simulink model "HANcoder_E407_TTA_Controller_v4_5"  (R2018b)
settings: Solver=FixedStepDiscrete  StartTime=0.0  StopTime=1  FixedStep=0.01  RelTol=1e-3
PreLoadFcn:
  | librarySetup
  | eval([bdroot,'_startup']) %Calling [modelName]_startup.m
values from neighbouring files (symbols this model uses):
  Backup_Board = 0    [HANcoder_E407_TTA_Controller_v3_5_startup.m]    (also in HANcoder_E407_TTA_Controller_v4_6_startup.m; HANcoder_E407_TTA_Controller_v4_7_startup.m; HANcoder_E407_TTA_Controller_v4_startup.m)
  basic_cycle_duration_bc0 = TM_Reset_Board   + COMP_duration    (= 212)    [HANcoder_E407_TTA_Controller_v3_5_startup.m]    (also in HANcoder_E407_TTA_Controller_v4_6_startup.m; HANcoder_E407_TTA_Controller_v4_7_startup.m; HANcoder_E407_TTA_Controller_v4_startup.m)
  basic_cycle_duration_bc1 = TM_Reset_Var_bc1 + COMP_duration    (= 288)    [HANcoder_E407_TTA_Controller_v3_5_startup.m]    (also in HANcoder_E407_TTA_Controller_v4_6_startup.m = 332; HANcoder_E407_TTA_Controller_v4_7_startup.m = 372; HANcoder_E407_TTA_Controller_v4_startup.m = 332)
  comm_delay_estimation1 = round(comm_delay_measured1*hardware_granularity/frequency_IRQ)    [HANcoder_E407_TTA_Controller_v3_5_startup.m]    (also in HANcoder_E407_TTA_Controller_v4_6_startup.m; HANcoder_E407_TTA_Controller_v4_7_startup.m; HANcoder_E407_TTA_Controller_v4_startup.m)
  comm_delay_estimation2 = round(comm_delay_measured2*hardware_granularity/frequency_IRQ)    [HANcoder_E407_TTA_Controller_v3_5_startup.m]    (also in HANcoder_E407_TTA_Controller_v4_6_startup.m; HANcoder_E407_TTA_Controller_v4_7_startup.m; HANcoder_E407_TTA_Controller_v4_startup.m)
  COMM_Period = 40    [HANcoder_E407_TTA_Controller_v3_5_startup.m]    (also in HANcoder_E407_TTA_Controller_v4_6_startup.m; HANcoder_E407_TTA_Controller_v4_7_startup.m; HANcoder_E407_TTA_Controller_v4_startup.m)
  COMM_Phase1 = Simulink.Parameter    [HANcoder_E407_TTA_Controller_v3_5_startup.m]    (also in HANcoder_E407_TTA_Controller_v4_6_startup.m; HANcoder_E407_TTA_Controller_v4_7_startup.m; HANcoder_E407_TTA_Controller_v4_startup.m)
  COMM_Phase2 = Simulink.Parameter    [HANcoder_E407_TTA_Controller_v3_5_startup.m]    (also in HANcoder_E407_TTA_Controller_v4_6_startup.m; HANcoder_E407_TTA_Controller_v4_7_startup.m; HANcoder_E407_TTA_Controller_v4_startup.m)
  COMM_Phase_init1 = Simulink.Parameter    [HANcoder_E407_TTA_Controller_v3_5_startup.m]    (also in HANcoder_E407_TTA_Controller_v4_6_startup.m; HANcoder_E407_TTA_Controller_v4_7_startup.m; HANcoder_E407_TTA_Controller_v4_startup.m)
  COMM_Phase_init2 = Simulink.Parameter    [HANcoder_E407_TTA_Controller_v3_5_startup.m]    (also in HANcoder_E407_TTA_Controller_v4_6_startup.m; HANcoder_E407_TTA_Controller_v4_7_startup.m; HANcoder_E407_TTA_Controller_v4_startup.m)
  COMP_duration = 4    [HANcoder_E407_TTA_Controller_v3_5_startup.m]    (also in HANcoder_E407_TTA_Controller_v4_6_startup.m; HANcoder_E407_TTA_Controller_v4_7_startup.m; HANcoder_E407_TTA_Controller_v4_startup.m)
  Controller1_Board = 1    [HANcoder_E407_TTA_Controller_v3_5_startup.m]    (also in HANcoder_E407_TTA_Controller_v4_6_startup.m; HANcoder_E407_TTA_Controller_v4_7_startup.m; HANcoder_E407_TTA_Controller_v4_startup.m)
  Controller2_Board = 2    [HANcoder_E407_TTA_Controller_v3_5_startup.m]    (also in HANcoder_E407_TTA_Controller_v4_6_startup.m; HANcoder_E407_TTA_Controller_v4_7_startup.m; HANcoder_E407_TTA_Controller_v4_startup.m)
  Controller3_Board = 3    [HANcoder_E407_TTA_Controller_v3_5_startup.m]    (also in HANcoder_E407_TTA_Controller_v4_6_startup.m; HANcoder_E407_TTA_Controller_v4_7_startup.m; HANcoder_E407_TTA_Controller_v4_startup.m)
  delta_a_set = Simulink.Parameter    [HANcoder_E407_TTA_Controller_v3_5_startup.m]    (also in HANcoder_E407_TTA_Controller_v4_6_startup.m; HANcoder_E407_TTA_Controller_v4_7_startup.m; HANcoder_E407_TTA_Controller_v4_startup.m)
  delta_f_set = Simulink.Parameter    [HANcoder_E407_TTA_Controller_v3_5_startup.m]    (also in HANcoder_E407_TTA_Controller_v4_6_startup.m; HANcoder_E407_TTA_Controller_v4_7_startup.m; HANcoder_E407_TTA_Controller_v4_startup.m)
  delta_max = 1    [HANcoder_E407_TTA_Controller_v3_5_startup.m]    (also in HANcoder_E407_TTA_Controller_v4_6_startup.m; HANcoder_E407_TTA_Controller_v4_7_startup.m; HANcoder_E407_TTA_Controller_v4_startup.m)
  delta_min = -1    [HANcoder_E407_TTA_Controller_v3_5_startup.m]    (also in HANcoder_E407_TTA_Controller_v4_6_startup.m; HANcoder_E407_TTA_Controller_v4_7_startup.m; HANcoder_E407_TTA_Controller_v4_startup.m)
  delta_precision = 6    [HANcoder_E407_TTA_Controller_v3_5_startup.m]    (also in HANcoder_E407_TTA_Controller_v4_6_startup.m; HANcoder_E407_TTA_Controller_v4_7_startup.m; HANcoder_E407_TTA_Controller_v4_startup.m)
  e_width = 0.1    [HANcoder_E407_TTA_Controller_v3_5_startup.m]    (also in HANcoder_E407_TTA_Controller_v4_6_startup.m; HANcoder_E407_TTA_Controller_v4_7_startup.m; HANcoder_E407_TTA_Controller_v4_startup.m)
  frequency_IRQ = 100    [HANcoder_E407_2xCAN_TEST_startup.m]    (also in HANcoder_E407_TTA_Controller_v3_5_startup.m; HANcoder_E407_TTA_Controller_v4_6_startup.m; HANcoder_E407_TTA_Controller_v4_7_startup.m; HANcoder_E407_TTA_Controller_v4_startup.m)
  HANtuneOverride = Simulink.Parameter    [HANcoder_E407_2xCAN_TEST_startup.m]    (also in HANcoder_E407_TTA_Controller_v3_5_startup.m; HANcoder_E407_TTA_Controller_v4_6_startup.m; HANcoder_E407_TTA_Controller_v4_7_startup.m; HANcoder_E407_TTA_Controller_v4_startup.m)
  hardware_granularity = 1000000    [HANcoder_E407_2xCAN_TEST_startup.m]    (also in HANcoder_E407_TTA_Controller_v3_5_startup.m; HANcoder_E407_TTA_Controller_v4_6_startup.m; HANcoder_E407_TTA_Controller_v4_7_startup.m; HANcoder_E407_TTA_Controller_v4_startup.m)
  I_a = 2.25    [HANcoder_E407_TTA_Controller_v3_5_startup.m]    (also in HANcoder_E407_TTA_Controller_v4_6_startup.m; HANcoder_E407_TTA_Controller_v4_7_startup.m; HANcoder_E407_TTA_Controller_v4_startup.m)
  I_f = 2.25    [HANcoder_E407_TTA_Controller_v3_5_startup.m]    (also in HANcoder_E407_TTA_Controller_v4_6_startup.m; HANcoder_E407_TTA_Controller_v4_7_startup.m; HANcoder_E407_TTA_Controller_v4_startup.m)
  idle_time_init = basic_cycle_duration_bc0 + basic_cycle_duration_bc1    (= 500)    [HANcoder_E407_TTA_Controller_v3_5_startup.m]    (also in HANcoder_E407_TTA_Controller_v4_6_startup.m = 544; HANcoder_E407_TTA_Controller_v4_7_startup.m = 584; HANcoder_E407_TTA_Controller_v4_startup.m = 544)
  Input_Gen_Board = 4    [HANcoder_E407_TTA_Controller_v3_5_startup.m]    (also in HANcoder_E407_TTA_Controller_v4_6_startup.m; HANcoder_E407_TTA_Controller_v4_7_startup.m; HANcoder_E407_TTA_Controller_v4_startup.m)
  LA_Clock_Gr = 1    [HANcoder_E407_TTA_Controller_v3_5_startup.m]    (also in HANcoder_E407_TTA_Controller_v4_6_startup.m; HANcoder_E407_TTA_Controller_v4_7_startup.m; HANcoder_E407_TTA_Controller_v4_startup.m)
  LA_COMM_dly = 1    [HANcoder_E407_TTA_Controller_v3_5_startup.m]    (also in HANcoder_E407_TTA_Controller_v4_6_startup.m; HANcoder_E407_TTA_Controller_v4_7_startup.m; HANcoder_E407_TTA_Controller_v4_startup.m)
  LA_COMM_Err = 1    [HANcoder_E407_TTA_Controller_v3_5_startup.m]    (also in HANcoder_E407_TTA_Controller_v4_6_startup.m; HANcoder_E407_TTA_Controller_v4_7_startup.m; HANcoder_E407_TTA_Controller_v4_startup.m)
  LA_E_Desync = 1    [HANcoder_E407_TTA_Controller_v3_5_startup.m]    (also in HANcoder_E407_TTA_Controller_v4_6_startup.m; HANcoder_E407_TTA_Controller_v4_7_startup.m; HANcoder_E407_TTA_Controller_v4_startup.m)
  LA_MEX_Flag = 1    [HANcoder_E407_TTA_Controller_v3_5_startup.m]    (also in HANcoder_E407_TTA_Controller_v4_6_startup.m; HANcoder_E407_TTA_Controller_v4_7_startup.m; HANcoder_E407_TTA_Controller_v4_startup.m)
  LA_Task_Act = 1    [HANcoder_E407_TTA_Controller_v3_5_startup.m]    (also in HANcoder_E407_TTA_Controller_v4_6_startup.m; HANcoder_E407_TTA_Controller_v4_7_startup.m; HANcoder_E407_TTA_Controller_v4_startup.m)
  m_v = 100.0    (= 100)    [HANcoder_E407_TTA_Controller_v3_5_startup.m]    (also in HANcoder_E407_TTA_Controller_v4_6_startup.m; HANcoder_E407_TTA_Controller_v4_7_startup.m; HANcoder_E407_TTA_Controller_v4_startup.m)
  Master_Role = 1    [HANcoder_E407_TTA_Controller_v3_5_startup.m]    (also in HANcoder_E407_TTA_Controller_v4_6_startup.m; HANcoder_E407_TTA_Controller_v4_7_startup.m; HANcoder_E407_TTA_Controller_v4_startup.m)
  matrix_cycle_duration = basic_cycle_duration_bc0 + basic_cycle_duration_bc1    (= 500)    [HANcoder_E407_TTA_Controller_v3_5_startup.m]    (also in HANcoder_E407_TTA_Controller_v4_6_startup.m = 544; HANcoder_E407_TTA_Controller_v4_7_startup.m = 584; HANcoder_E407_TTA_Controller_v4_startup.m = 544)
  matrix_rows = 2    [HANcoder_E407_TTA_Controller_v3_5_startup.m]    (also in HANcoder_E407_TTA_Controller_v4_6_startup.m; HANcoder_E407_TTA_Controller_v4_7_startup.m; HANcoder_E407_TTA_Controller_v4_startup.m)
  max_desync = 15    [HANcoder_E407_TTA_Controller_v3_5_startup.m]    (also in HANcoder_E407_TTA_Controller_v4_6_startup.m; HANcoder_E407_TTA_Controller_v4_7_startup.m = 30; HANcoder_E407_TTA_Controller_v4_startup.m)
  max_num_msgs_CAN1 = 2^Tx_bit_number-1    (= 7)    [HANcoder_E407_TTA_Controller_v3_5_startup.m]    (also in HANcoder_E407_TTA_Controller_v4_6_startup.m = 15; HANcoder_E407_TTA_Controller_v4_7_startup.m = 15; HANcoder_E407_TTA_Controller_v4_startup.m)
  max_num_msgs_CAN2 = max_num_msgs_CAN1    (= 7)    [HANcoder_E407_TTA_Controller_v3_5_startup.m]    (also in HANcoder_E407_TTA_Controller_v4_6_startup.m = 15; HANcoder_E407_TTA_Controller_v4_7_startup.m = 15; HANcoder_E407_TTA_Controller_v4_startup.m)
  min_desync = (-1)*max_desync    (= -15)    [HANcoder_E407_TTA_Controller_v3_5_startup.m]    (also in HANcoder_E407_TTA_Controller_v4_6_startup.m; HANcoder_E407_TTA_Controller_v4_7_startup.m = -30; HANcoder_E407_TTA_Controller_v4_startup.m)
  OutControl1_ID = 23    [HANcoder_E407_TTA_Controller_v3_5_startup.m]    (also in HANcoder_E407_TTA_Controller_v4_6_startup.m; HANcoder_E407_TTA_Controller_v4_7_startup.m; HANcoder_E407_TTA_Controller_v4_startup.m)
  OutControl2_ID = 24    [HANcoder_E407_TTA_Controller_v3_5_startup.m]    (also in HANcoder_E407_TTA_Controller_v4_6_startup.m; HANcoder_E407_TTA_Controller_v4_7_startup.m; HANcoder_E407_TTA_Controller_v4_startup.m)
  OutEmulator_ID = 25    [HANcoder_E407_TTA_Controller_v3_5_startup.m]    (also in HANcoder_E407_TTA_Controller_v4_6_startup.m = 26; HANcoder_E407_TTA_Controller_v4_7_startup.m = 26; HANcoder_E407_TTA_Controller_v4_startup.m)
  OutMaster_ID = 25    [HANcoder_E407_TTA_Controller_v4_6_startup.m]    (also in HANcoder_E407_TTA_Controller_v4_7_startup.m; HANcoder_E407_TTA_Controller_v4_startup.m = 26)
  R_al = 0.10    (= 0.1)    [HANcoder_E407_TTA_Controller_v3_5_startup.m]    (also in HANcoder_E407_TTA_Controller_v4_6_startup.m; HANcoder_E407_TTA_Controller_v4_7_startup.m; HANcoder_E407_TTA_Controller_v4_startup.m)
  R_ar = 0.10    (= 0.1)    [HANcoder_E407_TTA_Controller_v3_5_startup.m]    (also in HANcoder_E407_TTA_Controller_v4_6_startup.m; HANcoder_E407_TTA_Controller_v4_7_startup.m; HANcoder_E407_TTA_Controller_v4_startup.m)
  R_fl = 0.10    (= 0.1)    [HANcoder_E407_TTA_Controller_v3_5_startup.m]    (also in HANcoder_E407_TTA_Controller_v4_6_startup.m; HANcoder_E407_TTA_Controller_v4_7_startup.m; HANcoder_E407_TTA_Controller_v4_startup.m)
  R_fr = 0.10    (= 0.1)    [HANcoder_E407_TTA_Controller_v3_5_startup.m]    (also in HANcoder_E407_TTA_Controller_v4_6_startup.m; HANcoder_E407_TTA_Controller_v4_7_startup.m; HANcoder_E407_TTA_Controller_v4_startup.m)
  script_run = Simulink.Parameter    [HANcoder_E407_TTA_Controller_v3_5_startup.m]    (also in HANcoder_E407_TTA_Controller_v4_6_startup.m; HANcoder_E407_TTA_Controller_v4_7_startup.m; HANcoder_E407_TTA_Controller_v4_startup.m)
  SensorValues_ID = 22    [HANcoder_E407_TTA_Controller_v3_5_startup.m]    (also in HANcoder_E407_TTA_Controller_v4_6_startup.m; HANcoder_E407_TTA_Controller_v4_7_startup.m; HANcoder_E407_TTA_Controller_v4_startup.m)
  SetValues_ID = 21    [HANcoder_E407_TTA_Controller_v3_5_startup.m]    (also in HANcoder_E407_TTA_Controller_v4_6_startup.m; HANcoder_E407_TTA_Controller_v4_7_startup.m; HANcoder_E407_TTA_Controller_v4_startup.m)
  Slave_Role = 2    [HANcoder_E407_TTA_Controller_v3_5_startup.m]    (also in HANcoder_E407_TTA_Controller_v4_6_startup.m; HANcoder_E407_TTA_Controller_v4_7_startup.m; HANcoder_E407_TTA_Controller_v4_startup.m)
  speed_k_d = Simulink.Parameter    [HANcoder_E407_TTA_Controller_v3_5_startup.m]    (also in HANcoder_E407_TTA_Controller_v4_6_startup.m; HANcoder_E407_TTA_Controller_v4_7_startup.m; HANcoder_E407_TTA_Controller_v4_startup.m)
  speed_k_i = Simulink.Parameter    [HANcoder_E407_TTA_Controller_v3_5_startup.m]    (also in HANcoder_E407_TTA_Controller_v4_6_startup.m; HANcoder_E407_TTA_Controller_v4_7_startup.m; HANcoder_E407_TTA_Controller_v4_startup.m)
  speed_k_p = Simulink.Parameter    [HANcoder_E407_TTA_Controller_v3_5_startup.m]    (also in HANcoder_E407_TTA_Controller_v4_6_startup.m; HANcoder_E407_TTA_Controller_v4_7_startup.m; HANcoder_E407_TTA_Controller_v4_startup.m)
  speed_max = 10    [HANcoder_E407_TTA_Controller_v3_5_startup.m]    (also in HANcoder_E407_TTA_Controller_v4_6_startup.m; HANcoder_E407_TTA_Controller_v4_7_startup.m; HANcoder_E407_TTA_Controller_v4_startup.m)
  speed_min = -10    [HANcoder_E407_TTA_Controller_v3_5_startup.m]    (also in HANcoder_E407_TTA_Controller_v4_6_startup.m; HANcoder_E407_TTA_Controller_v4_7_startup.m; HANcoder_E407_TTA_Controller_v4_startup.m)
  speed_precision = 3    [HANcoder_E407_TTA_Controller_v3_5_startup.m]    (also in HANcoder_E407_TTA_Controller_v4_6_startup.m; HANcoder_E407_TTA_Controller_v4_7_startup.m; HANcoder_E407_TTA_Controller_v4_startup.m)
  Sync_ID = 1    [HANcoder_E407_TTA_Controller_v3_5_startup.m]    (also in HANcoder_E407_TTA_Controller_v4_6_startup.m; HANcoder_E407_TTA_Controller_v4_7_startup.m; HANcoder_E407_TTA_Controller_v4_startup.m)
  tau_max = 5    [HANcoder_E407_TTA_Controller_v3_5_startup.m]    (also in HANcoder_E407_TTA_Controller_v4_6_startup.m; HANcoder_E407_TTA_Controller_v4_7_startup.m; HANcoder_E407_TTA_Controller_v4_startup.m)
  tau_min = -5    [HANcoder_E407_TTA_Controller_v3_5_startup.m]    (also in HANcoder_E407_TTA_Controller_v4_6_startup.m; HANcoder_E407_TTA_Controller_v4_7_startup.m; HANcoder_E407_TTA_Controller_v4_startup.m)
  tau_range = abs(tau_max) + abs(tau_min)    [HANcoder_E407_TTA_Controller_v3_5_startup.m]    (also in HANcoder_E407_TTA_Controller_v4_6_startup.m; HANcoder_E407_TTA_Controller_v4_7_startup.m; HANcoder_E407_TTA_Controller_v4_startup.m)
  theta_max = (speed_max/R_fr)*matrix_cycle_duration*frequency_IRQ/hardware_granularity    (= 5)    [HANcoder_E407_TTA_Controller_v3_5_startup.m]    (also in HANcoder_E407_TTA_Controller_v4_6_startup.m = 5.44; HANcoder_E407_TTA_Controller_v4_7_startup.m = 5.84; HANcoder_E407_TTA_Controller_v4_startup.m = 5.44)
  theta_min = (-1)*theta_max    (= -5)    [HANcoder_E407_TTA_Controller_v3_5_startup.m]    (also in HANcoder_E407_TTA_Controller_v4_6_startup.m = -5.44; HANcoder_E407_TTA_Controller_v4_7_startup.m = -5.84; HANcoder_E407_TTA_Controller_v4_startup.m = -5.44)
  theta_precision = 7-(fix(log2(theta_max))+1)    [HANcoder_E407_TTA_Controller_v3_5_startup.m]    (also in HANcoder_E407_TTA_Controller_v4_6_startup.m; HANcoder_E407_TTA_Controller_v4_7_startup.m; HANcoder_E407_TTA_Controller_v4_startup.m)
  Tl_a = 0.6    [HANcoder_E407_TTA_Controller_v3_5_startup.m]    (also in HANcoder_E407_TTA_Controller_v4_6_startup.m; HANcoder_E407_TTA_Controller_v4_7_startup.m; HANcoder_E407_TTA_Controller_v4_startup.m)
  Tl_f = 0.6    [HANcoder_E407_TTA_Controller_v3_5_startup.m]    (also in HANcoder_E407_TTA_Controller_v4_6_startup.m; HANcoder_E407_TTA_Controller_v4_7_startup.m; HANcoder_E407_TTA_Controller_v4_startup.m)
  TM_Check_Output_Control1 = TM_COMM_Output_Control1 + COMM_duration    (= 188)    [HANcoder_E407_TTA_Controller_v3_5_startup.m]    (also in HANcoder_E407_TTA_Controller_v4_6_startup.m; HANcoder_E407_TTA_Controller_v4_7_startup.m; HANcoder_E407_TTA_Controller_v4_startup.m)
  TM_Check_Output_Control2 = TM_COMM_Output_Control2 + COMM_duration    (= 232)    [HANcoder_E407_TTA_Controller_v3_5_startup.m]    (also in HANcoder_E407_TTA_Controller_v4_6_startup.m; HANcoder_E407_TTA_Controller_v4_7_startup.m; HANcoder_E407_TTA_Controller_v4_startup.m)
  TM_Check_Output_Emulator = TM_COMM_Output_Emulator + COMM_duration    (= 280)    [HANcoder_E407_TTA_Controller_v3_5_startup.m]    (also in HANcoder_E407_TTA_Controller_v4_6_startup.m = 320; HANcoder_E407_TTA_Controller_v4_7_startup.m = 360; HANcoder_E407_TTA_Controller_v4_startup.m = 320)
  TM_Check_Output_Emulator_2 = TM_Check_Output_Emulator + 2    (= 282)    [HANcoder_E407_TTA_Controller_v3_5_startup.m]    (also in HANcoder_E407_TTA_Controller_v4_6_startup.m = 322; HANcoder_E407_TTA_Controller_v4_7_startup.m = 362; HANcoder_E407_TTA_Controller_v4_startup.m = 322)
  TM_Check_Output_Emulator_3 = TM_Check_Output_Emulator_2 + 2    (= 324)    [HANcoder_E407_TTA_Controller_v4_6_startup.m]    (also in HANcoder_E407_TTA_Controller_v4_7_startup.m = 364; HANcoder_E407_TTA_Controller_v4_startup.m)
  TM_Check_Sensor_Values = TM_COMM_Sensor_Values + COMM_duration    (= 132)    [HANcoder_E407_TTA_Controller_v3_5_startup.m]    (also in HANcoder_E407_TTA_Controller_v4_6_startup.m; HANcoder_E407_TTA_Controller_v4_7_startup.m; HANcoder_E407_TTA_Controller_v4_startup.m)
  TM_Check_Sensor_Values_2 = TM_Check_Sensor_Values + 2    (= 134)    [HANcoder_E407_TTA_Controller_v3_5_startup.m]    (also in HANcoder_E407_TTA_Controller_v4_6_startup.m; HANcoder_E407_TTA_Controller_v4_7_startup.m; HANcoder_E407_TTA_Controller_v4_startup.m)
  TM_Check_Set_Values = TM_COMM_Set_Values + COMM_duration    (= 88)    [HANcoder_E407_TTA_Controller_v3_5_startup.m]    (also in HANcoder_E407_TTA_Controller_v4_6_startup.m; HANcoder_E407_TTA_Controller_v4_7_startup.m; HANcoder_E407_TTA_Controller_v4_startup.m)
  TM_Check_Set_Values_2 = TM_Check_Set_Values + 2    (= 90)    [HANcoder_E407_TTA_Controller_v3_5_startup.m]    (also in HANcoder_E407_TTA_Controller_v4_6_startup.m; HANcoder_E407_TTA_Controller_v4_7_startup.m; HANcoder_E407_TTA_Controller_v4_startup.m)
  TM_Check_Sync = TM_COMM_Sync   + COMM_duration    (= 40)    [HANcoder_E407_TTA_Controller_v3_5_startup.m]    (also in HANcoder_E407_TTA_Controller_v4_6_startup.m; HANcoder_E407_TTA_Controller_v4_7_startup.m; HANcoder_E407_TTA_Controller_v4_startup.m)
  TM_Check_TOuts = TM_Count_Vote3 + COMP_duration    (= 196)    [HANcoder_E407_TTA_Controller_v3_5_startup.m]    (also in HANcoder_E407_TTA_Controller_v4_6_startup.m; HANcoder_E407_TTA_Controller_v4_7_startup.m; HANcoder_E407_TTA_Controller_v4_startup.m)
  TM_Check_Vote1 = TM_COMM_Vote1  + COMM_duration    (= 92)    [HANcoder_E407_TTA_Controller_v3_5_startup.m]    (also in HANcoder_E407_TTA_Controller_v4_6_startup.m; HANcoder_E407_TTA_Controller_v4_7_startup.m; HANcoder_E407_TTA_Controller_v4_startup.m)
  TM_Check_Vote2 = TM_COMM_Vote2  + COMM_duration    (= 140)    [HANcoder_E407_TTA_Controller_v3_5_startup.m]    (also in HANcoder_E407_TTA_Controller_v4_6_startup.m; HANcoder_E407_TTA_Controller_v4_7_startup.m; HANcoder_E407_TTA_Controller_v4_startup.m)
  TM_Check_Vote2_2 = TM_Check_Vote2 + 2    (= 142)    [HANcoder_E407_TTA_Controller_v3_5_startup.m]    (also in HANcoder_E407_TTA_Controller_v4_6_startup.m; HANcoder_E407_TTA_Controller_v4_7_startup.m; HANcoder_E407_TTA_Controller_v4_startup.m)
  TM_Check_Vote3 = TM_COMM_Vote3  + COMM_duration    (= 188)    [HANcoder_E407_TTA_Controller_v3_5_startup.m]    (also in HANcoder_E407_TTA_Controller_v4_6_startup.m; HANcoder_E407_TTA_Controller_v4_7_startup.m; HANcoder_E407_TTA_Controller_v4_startup.m)
  TM_COMM_Output_Control1 = TM_Velocity + COMP_duration    (= 148)    [HANcoder_E407_TTA_Controller_v3_5_startup.m]    (also in HANcoder_E407_TTA_Controller_v4_6_startup.m; HANcoder_E407_TTA_Controller_v4_7_startup.m; HANcoder_E407_TTA_Controller_v4_startup.m)
  TM_COMM_Output_Control2 = TM_Check_Output_Control1 + COMP_duration    (= 192)    [HANcoder_E407_TTA_Controller_v3_5_startup.m]    (also in HANcoder_E407_TTA_Controller_v4_6_startup.m; HANcoder_E407_TTA_Controller_v4_7_startup.m; HANcoder_E407_TTA_Controller_v4_startup.m)
  TM_COMM_Output_Emulator = TM_TMR + COMP_duration    (= 240)    [HANcoder_E407_TTA_Controller_v3_5_startup.m]    (also in HANcoder_E407_TTA_Controller_v4_6_startup.m = 280; HANcoder_E407_TTA_Controller_v4_7_startup.m = 320; HANcoder_E407_TTA_Controller_v4_startup.m = 280)
  TM_COMM_Output_Master = TM_Check_Output_Control2 + COMM_duration    (= 272)    [HANcoder_E407_TTA_Controller_v4_6_startup.m]    (also in HANcoder_E407_TTA_Controller_v4_7_startup.m; HANcoder_E407_TTA_Controller_v4_startup.m)
  TM_COMM_Sensor_Values = TM_Check_Set_Values + COMP_duration    (= 92)    [HANcoder_E407_TTA_Controller_v3_5_startup.m]    (also in HANcoder_E407_TTA_Controller_v4_6_startup.m; HANcoder_E407_TTA_Controller_v4_7_startup.m; HANcoder_E407_TTA_Controller_v4_startup.m)
  TM_COMM_Set_Values = TM_Update_LT + COMP_duration    (= 48)    [HANcoder_E407_TTA_Controller_v3_5_startup.m]    (also in HANcoder_E407_TTA_Controller_v4_6_startup.m; HANcoder_E407_TTA_Controller_v4_7_startup.m; HANcoder_E407_TTA_Controller_v4_startup.m)
  TM_COMM_Sync = basic_cycle_start    (= 0)    [HANcoder_E407_TTA_Controller_v3_5_startup.m]    (also in HANcoder_E407_TTA_Controller_v4_6_startup.m; HANcoder_E407_TTA_Controller_v4_7_startup.m; HANcoder_E407_TTA_Controller_v4_startup.m)
  TM_COMM_Vote1 = TM_Vote_Dec    + COMP_duration    (= 52)    [HANcoder_E407_TTA_Controller_v3_5_startup.m]    (also in HANcoder_E407_TTA_Controller_v4_6_startup.m; HANcoder_E407_TTA_Controller_v4_7_startup.m; HANcoder_E407_TTA_Controller_v4_startup.m)
  TM_COMM_Vote2 = TM_Count_Vote1 + COMP_duration    (= 100)    [HANcoder_E407_TTA_Controller_v3_5_startup.m]    (also in HANcoder_E407_TTA_Controller_v4_6_startup.m; HANcoder_E407_TTA_Controller_v4_7_startup.m; HANcoder_E407_TTA_Controller_v4_startup.m)
  TM_COMM_Vote3 = TM_Count_Vote2 + COMP_duration    (= 148)    [HANcoder_E407_TTA_Controller_v3_5_startup.m]    (also in HANcoder_E407_TTA_Controller_v4_6_startup.m; HANcoder_E407_TTA_Controller_v4_7_startup.m; HANcoder_E407_TTA_Controller_v4_startup.m)
  TM_Count_Vote1 = TM_Check_Vote1 + COMP_duration    (= 96)    [HANcoder_E407_TTA_Controller_v3_5_startup.m]    (also in HANcoder_E407_TTA_Controller_v4_6_startup.m; HANcoder_E407_TTA_Controller_v4_7_startup.m; HANcoder_E407_TTA_Controller_v4_startup.m)
  TM_Count_Vote2 = TM_Check_Vote2 + COMP_duration    (= 144)    [HANcoder_E407_TTA_Controller_v3_5_startup.m]    (also in HANcoder_E407_TTA_Controller_v4_6_startup.m; HANcoder_E407_TTA_Controller_v4_7_startup.m; HANcoder_E407_TTA_Controller_v4_startup.m)
  TM_Count_Vote3 = TM_Check_Vote3 + COMP_duration    (= 192)    [HANcoder_E407_TTA_Controller_v3_5_startup.m]    (also in HANcoder_E407_TTA_Controller_v4_6_startup.m; HANcoder_E407_TTA_Controller_v4_7_startup.m; HANcoder_E407_TTA_Controller_v4_startup.m)
  TM_Data_bc0 = TM_COMM_Sync    (= 0)    [HANcoder_E407_TTA_Controller_v3_5_startup.m]    (also in HANcoder_E407_TTA_Controller_v4_6_startup.m; HANcoder_E407_TTA_Controller_v4_7_startup.m; HANcoder_E407_TTA_Controller_v4_startup.m)
  TM_Data_bc1 = TM_Data_bc0(1:4)    [HANcoder_E407_TTA_Controller_v3_5_startup.m]    (also in HANcoder_E407_TTA_Controller_v4_6_startup.m; HANcoder_E407_TTA_Controller_v4_7_startup.m; HANcoder_E407_TTA_Controller_v4_startup.m)
  TM_New_Master = TM_Check_TOuts + COMP_duration    (= 200)    [HANcoder_E407_TTA_Controller_v3_5_startup.m]    (also in HANcoder_E407_TTA_Controller_v4_6_startup.m; HANcoder_E407_TTA_Controller_v4_7_startup.m; HANcoder_E407_TTA_Controller_v4_startup.m)
  TM_Reset_Board = TM_Reset_Var   + COMP_duration    (= 208)    [HANcoder_E407_TTA_Controller_v3_5_startup.m]    (also in HANcoder_E407_TTA_Controller_v4_6_startup.m; HANcoder_E407_TTA_Controller_v4_7_startup.m; HANcoder_E407_TTA_Controller_v4_startup.m)
  TM_Reset_Var = TM_New_Master  + COMP_duration    (= 204)    [HANcoder_E407_TTA_Controller_v3_5_startup.m]    (also in HANcoder_E407_TTA_Controller_v4_6_startup.m; HANcoder_E407_TTA_Controller_v4_7_startup.m; HANcoder_E407_TTA_Controller_v4_startup.m)
  TM_Reset_Var_bc1 = TM_Check_Output_Emulator + COMP_duration    (= 284)    [HANcoder_E407_TTA_Controller_v3_5_startup.m]    (also in HANcoder_E407_TTA_Controller_v4_6_startup.m = 328; HANcoder_E407_TTA_Controller_v4_7_startup.m = 368; HANcoder_E407_TTA_Controller_v4_startup.m = 328)
  TM_Reset_Var_bc1_2 = TM_Reset_Var_bc1 + 2    (= 286)    [HANcoder_E407_TTA_Controller_v3_5_startup.m]    (also in HANcoder_E407_TTA_Controller_v4_6_startup.m = 330; HANcoder_E407_TTA_Controller_v4_7_startup.m = 370; HANcoder_E407_TTA_Controller_v4_startup.m = 330)
  TM_Steer = TM_Check_Sensor_Values + COMP_duration    (= 136)    [HANcoder_E407_TTA_Controller_v3_5_startup.m]    (also in HANcoder_E407_TTA_Controller_v4_6_startup.m; HANcoder_E407_TTA_Controller_v4_7_startup.m; HANcoder_E407_TTA_Controller_v4_startup.m)
  TM_TMR = TM_Check_Output_Control2 + COMP_duration    (= 236)    [HANcoder_E407_TTA_Controller_v3_5_startup.m]    (also in HANcoder_E407_TTA_Controller_v4_6_startup.m = 276; HANcoder_E407_TTA_Controller_v4_7_startup.m = 316; HANcoder_E407_TTA_Controller_v4_startup.m = 276)
  TM_TMR_2 = TM_TMR + 1    (= 237)    [HANcoder_E407_TTA_Controller_v3_5_startup.m]    (also in HANcoder_E407_TTA_Controller_v4_6_startup.m = 277; HANcoder_E407_TTA_Controller_v4_7_startup.m = 317; HANcoder_E407_TTA_Controller_v4_startup.m = 277)
  TM_TMR_3 = TM_TMR + 3    (= 239)    [HANcoder_E407_TTA_Controller_v3_5_startup.m]    (also in HANcoder_E407_TTA_Controller_v4_6_startup.m = 279; HANcoder_E407_TTA_Controller_v4_7_startup.m = 319; HANcoder_E407_TTA_Controller_v4_startup.m = 279)
  TM_Torque = TM_Steer + COMP_duration    (= 140)    [HANcoder_E407_TTA_Controller_v3_5_startup.m]    (also in HANcoder_E407_TTA_Controller_v4_6_startup.m; HANcoder_E407_TTA_Controller_v4_7_startup.m; HANcoder_E407_TTA_Controller_v4_startup.m)
  TM_Type_bc0 = COMM    (= 0)    [HANcoder_E407_TTA_Controller_v3_5_startup.m]    (also in HANcoder_E407_TTA_Controller_v4_6_startup.m; HANcoder_E407_TTA_Controller_v4_7_startup.m; HANcoder_E407_TTA_Controller_v4_startup.m)
  TM_Type_bc1 = TM_Type_bc0(1:4)    [HANcoder_E407_TTA_Controller_v3_5_startup.m]    (also in HANcoder_E407_TTA_Controller_v4_6_startup.m; HANcoder_E407_TTA_Controller_v4_7_startup.m; HANcoder_E407_TTA_Controller_v4_startup.m)
  TM_Update_LT = TM_Check_Sync  + COMP_duration    (= 44)    [HANcoder_E407_TTA_Controller_v3_5_startup.m]    (also in HANcoder_E407_TTA_Controller_v4_6_startup.m; HANcoder_E407_TTA_Controller_v4_7_startup.m; HANcoder_E407_TTA_Controller_v4_startup.m)
  TM_Update_LT_2 = TM_Update_LT   + 2    (= 46)    [HANcoder_E407_TTA_Controller_v3_5_startup.m]    (also in HANcoder_E407_TTA_Controller_v4_6_startup.m; HANcoder_E407_TTA_Controller_v4_7_startup.m; HANcoder_E407_TTA_Controller_v4_startup.m)
  TM_Velocity = TM_Torque + COMP_duration    (= 144)    [HANcoder_E407_TTA_Controller_v3_5_startup.m]    (also in HANcoder_E407_TTA_Controller_v4_6_startup.m; HANcoder_E407_TTA_Controller_v4_7_startup.m; HANcoder_E407_TTA_Controller_v4_startup.m)
  TM_Vote_Dec = TM_Update_LT   + COMP_duration    (= 48)    [HANcoder_E407_TTA_Controller_v3_5_startup.m]    (also in HANcoder_E407_TTA_Controller_v4_6_startup.m; HANcoder_E407_TTA_Controller_v4_7_startup.m; HANcoder_E407_TTA_Controller_v4_startup.m)
  TM_Vote_Dec_2 = TM_Vote_Dec    + 2    (= 50)    [HANcoder_E407_TTA_Controller_v3_5_startup.m]    (also in HANcoder_E407_TTA_Controller_v4_6_startup.m; HANcoder_E407_TTA_Controller_v4_7_startup.m; HANcoder_E407_TTA_Controller_v4_startup.m)
  torque_a_k_d = Simulink.Parameter    [HANcoder_E407_TTA_Controller_v3_5_startup.m]    (also in HANcoder_E407_TTA_Controller_v4_6_startup.m; HANcoder_E407_TTA_Controller_v4_7_startup.m; HANcoder_E407_TTA_Controller_v4_startup.m)
  torque_a_k_i = Simulink.Parameter    [HANcoder_E407_TTA_Controller_v3_5_startup.m]    (also in HANcoder_E407_TTA_Controller_v4_6_startup.m; HANcoder_E407_TTA_Controller_v4_7_startup.m; HANcoder_E407_TTA_Controller_v4_startup.m)
  torque_a_k_p = Simulink.Parameter    [HANcoder_E407_TTA_Controller_v3_5_startup.m]    (also in HANcoder_E407_TTA_Controller_v4_6_startup.m; HANcoder_E407_TTA_Controller_v4_7_startup.m; HANcoder_E407_TTA_Controller_v4_startup.m)
  torque_f_k_d = Simulink.Parameter    [HANcoder_E407_TTA_Controller_v3_5_startup.m]    (also in HANcoder_E407_TTA_Controller_v4_6_startup.m; HANcoder_E407_TTA_Controller_v4_7_startup.m; HANcoder_E407_TTA_Controller_v4_startup.m)
  torque_f_k_i = Simulink.Parameter    [HANcoder_E407_TTA_Controller_v3_5_startup.m]    (also in HANcoder_E407_TTA_Controller_v4_6_startup.m; HANcoder_E407_TTA_Controller_v4_7_startup.m; HANcoder_E407_TTA_Controller_v4_startup.m)
  ... (+7 more)
undefined symbols (not defined in the file or in its folder): A0, A1, A2, A3, A4, CON2, CON3, CON4, D10, D12, D13, D2, D3, D8, D9
libraries: hdlsllib x467, HANcoder_STM32_Target x30, simulink x3, simulink_extras x1
(part 74 of 80)

== system HANcoder_E407_TTA_Controller_v4_5/HANcoder STM32 Target - E407-STM32 algorithm/TTA CAN System/TTA System/Matrix Cycle Manager/Input Generator Matrix Cycle/input generator basic cycle 1/COMP Task - Sync bc1 check/Process_Messages/Demux message CAN1 and check coherence/msg_count>2_DEBUG ==
  note: If this board received during this COMM a message
      | with a count greater than 1, it means the first message
      | sent was missed, but at least one later msg reached
      | this board.
  msg_c : Inport
  Constant : Constant
  Constant1 : Constant
  Data Store Read : DataStoreRead  DataStoreName=msg_count_DEBUG
  Data Store Read1 : DataStoreRead  DataStoreName=msg_count_DEBUG
  Data Store Write : DataStoreWrite  DataStoreName=msg_count_DEBUG
  GreaterThan : RelationalOperator  Operator=>  OutDataTypeStr=boolean  RndMeth=Simplest
  Plus : Sum
  Switch : Switch  Criteria=u2 > Threshold
  wires:
  Constant1/1 -> GreaterThan/2
  GreaterThan/1 -> Switch/2
  Switch/1 -> Data Store Write/1
  Constant/1 -> Plus/2
  Data Store Read1/1 -> Plus/1
  Plus/1 -> Switch/1
  Data Store Read/1 -> Switch/3
  msg_c/1 -> GreaterThan/1

== system HANcoder_E407_TTA_Controller_v4_5/HANcoder STM32 Target - E407-STM32 algorithm/TTA CAN System/TTA System/Matrix Cycle Manager/Input Generator Matrix Cycle/input generator basic cycle 1/COMP Task - Sync bc1 check/Process_Messages/Demux message CAN1 and check coherence1/Subsystem ==
  Msg_Temporal_Data : Inport
  Bit Shift : hdlsllib/Logic and Bit Operations/Bit Shift  mode=Shift Right Logical  N=7
      settings: SourceProductName=HDL Coder  SourceProductBaseCode=HD
  Bit Shift1 : hdlsllib/Logic and Bit Operations/Bit Shift  mode=Shift Right Logical  N=5
      settings: SourceProductName=HDL Coder  SourceProductBaseCode=HD
  Bit Shift2 : hdlsllib/Logic and Bit Operations/Bit Shift  mode=Shift Right Logical  N=4
      settings: SourceProductName=HDL Coder  SourceProductBaseCode=HD
  Bit Shift3 : hdlsllib/Logic and Bit Operations/Bit Shift  mode=Shift Left Logical  N=1
      settings: SourceProductName=HDL Coder  SourceProductBaseCode=HD
  Bit Shift4 : hdlsllib/Logic and Bit Operations/Bit Shift  mode=Shift Left Logical  N=4
      settings: SourceProductName=HDL Coder  SourceProductBaseCode=HD
  basic_cycle : Outport
  msg_count : Outport  Port=2
  board_id : Outport  Port=3
  wires:
  Bit Shift4/1 -> Bit Shift2/1
  Bit Shift3/1 -> Bit Shift1/1
  Bit Shift2/1 -> board_id/1
  Bit Shift1/1 -> msg_count/1
  Msg_Temporal_Data/1 -> Bit Shift3/1, Bit Shift/1, Bit Shift4/1
  Bit Shift/1 -> basic_cycle/1

== system HANcoder_E407_TTA_Controller_v4_5/HANcoder STM32 Target - E407-STM32 algorithm/TTA CAN System/TTA System/Matrix Cycle Manager/Input Generator Matrix Cycle/input generator basic cycle 1/COMP Task - Sync bc1 check/Process_Messages/Demux message CAN1 and check coherence1/msg_count>2_DEBUG ==
  note: If this board received during this COMM a message
      | with a count greater than 1, it means the first message
      | sent was missed, but at least one later msg reached
      | this board.
  msg_c : Inport
  Constant : Constant
  Constant1 : Constant
  Data Store Read : DataStoreRead  DataStoreName=msg_count_DEBUG
  Data Store Read1 : DataStoreRead  DataStoreName=msg_count_DEBUG
  Data Store Write : DataStoreWrite  DataStoreName=msg_count_DEBUG
  GreaterThan : RelationalOperator  Operator=>  OutDataTypeStr=boolean  RndMeth=Simplest
  Plus : Sum
  Switch : Switch  Criteria=u2 > Threshold
  wires:
  Constant1/1 -> GreaterThan/2
  GreaterThan/1 -> Switch/2
  Switch/1 -> Data Store Write/1
  Constant/1 -> Plus/2
  Data Store Read1/1 -> Plus/1
  Plus/1 -> Switch/1
  Data Store Read/1 -> Switch/3
  msg_c/1 -> GreaterThan/1

== system HANcoder_E407_TTA_Controller_v4_5/HANcoder STM32 Target - E407-STM32 algorithm/TTA CAN System/TTA System/Matrix Cycle Manager/Vehicle Emulator Matrix Cycle/vehicle emulator basic cycle 0/COMM Task - Sync bc 0/Transmission subtasks/Check msg transmission CAN1/TX buffer update CAN1 ==
  note: Transmission end - Set message to send through CAN 1
  note: Message Temporal Data
      |    Every message sends
      |    BasicCycle, Tx count
      |    and Verification msg
      |    as data
  note: Transmission ID
      |    Sync Msg: 1
      |    Vote Node 1: 11
      |    Vote Node 2: 12
      |    Vote Node 3: 13
  Tx_ID : Inport
  Msg_Value_Data : Inport  Port=2
  Enable : EnablePort
  Bus Selector : BusSelector  OutputSignals=signal2,signal3,signal4,signal5,signal6,signal7,signal8
  Cast : DataTypeConversion  OutDataTypeStr=uint32
  Cast1 : DataTypeConversion  OutDataTypeStr=uint8
  Cast16 : DataTypeConversion  OutDataTypeStr=uint8
  Cast4 : DataTypeConversion  OutDataTypeStr=uint8
  Data Store Read : DataStoreRead  Priority=50  DataStoreName=Tx_msg_count_CAN1
  Data Store Read1 : DataStoreRead  DataStoreName=Board_ID
  Data Store Read3 : DataStoreRead  DataStoreName=basic_cycle_count
  Data Store Write10 : DataStoreWrite  DataStoreName=Msg_Tx_CAN1  DataStoreElements=Msg_Tx_CAN1.Buffer_1#Msg_Tx_CAN1.Buffer_2#Msg_Tx_CAN1.Buffer_3#Msg_Tx_CAN1.Buffer_4#Msg_Tx_CAN1.Buffer_5#Msg_Tx_CAN1.Buffer_6#Msg_Tx_CAN1.Buffer_7#Msg_Tx_CAN1.Buffer_8
  Data Store Write8 : DataStoreWrite  DataStoreName=TxID_CAN1
  Msg_Data_Encoder : Subsystem
  wires:
  Cast/1 -> Data Store Write8/1
  Data Store Read3/1 -> Cast4/1
  Cast4/1 -> Msg_Data_Encoder/1(basic_cycle)
  Msg_Value_Data/1 -> Bus Selector/1
  Tx_ID/1 -> Cast/1
  Data Store Read/1 -> Cast1/1
  Cast16/1 -> Msg_Data_Encoder/3(board_number)
  Cast1/1 -> Msg_Data_Encoder/2(tx_counter)
  Data Store Read1/1 -> Cast16/1
  Msg_Data_Encoder/1(encoded_msg) -> Data Store Write10/1
  Bus Selector/1 -> Data Store Write10/2  "<signal2>"
  Bus Selector/2 -> Data Store Write10/3  "<signal3>"
  Bus Selector/3 -> Data Store Write10/4  "<signal4>"
  Bus Selector/4 -> Data Store Write10/5  "<signal5>"
  Bus Selector/5 -> Data Store Write10/6  "<signal6>"
  Bus Selector/6 -> Data Store Write10/7  "<signal7>"
  Bus Selector/7 -> Data Store Write10/8  "<signal8>"

== system HANcoder_E407_TTA_Controller_v4_5/HANcoder STM32 Target - E407-STM32 algorithm/TTA CAN System/TTA System/Matrix Cycle Manager/Vehicle Emulator Matrix Cycle/vehicle emulator basic cycle 0/COMM Task - Sync bc 0/Transmission subtasks/Check msg transmission CAN2/TX buffer update CAN2 ==
  note: Transmission end - Set message to send through CAN
  note: Transmission ID
      |    Sync Msg: 1
      |    Vote Node 1: 11
      |    Vote Node 2: 12
      |    Vote Node 3: 13
  note: Message Data
      |    Every message sends
      |    BasicCycle, Tx count
      |    and Verification msg
      |    as data
  Tx_ID : Inport
  Msg_Value_Data : Inport  Port=2
  Enable : EnablePort
  Bus Selector : BusSelector  OutputSignals=signal2,signal3,signal4,signal5,signal6,signal7,signal8
  Cast17 : DataTypeConversion  OutDataTypeStr=uint8
  Cast18 : DataTypeConversion  OutDataTypeStr=uint8
  Cast8 : DataTypeConversion  OutDataTypeStr=uint32
  Cast9 : DataTypeConversion  OutDataTypeStr=uint8
  Data Store Read : DataStoreRead  DataStoreName=Board_ID
  Data Store Read1 : DataStoreRead  Priority=50  DataStoreName=Tx_msg_count_CAN2
  Data Store Read6 : DataStoreRead  DataStoreName=basic_cycle_count
  Data Store Write4 : DataStoreWrite  DataStoreName=Msg_Tx_CAN2  DataStoreElements=Msg_Tx_CAN2.Buffer_1#Msg_Tx_CAN2.Buffer_2#Msg_Tx_CAN2.Buffer_3#Msg_Tx_CAN2.Buffer_4#Msg_Tx_CAN2.Buffer_5#Msg_Tx_CAN2.Buffer_6#Msg_Tx_CAN2.Buffer_7#Msg_Tx_CAN2.Buffer_8
  Data Store Write5 : DataStoreWrite  DataStoreName=TxID_CAN2
  Msg_Data_Encoder : Subsystem
  wires:
  Bus Selector/7 -> Data Store Write4/8  "<signal8>"
  Bus Selector/6 -> Data Store Write4/7  "<signal7>"
  Bus Selector/5 -> Data Store Write4/6  "<signal6>"
  Bus Selector/4 -> Data Store Write4/5  "<signal5>"
  Bus Selector/3 -> Data Store Write4/4  "<signal4>"
  Bus Selector/2 -> Data Store Write4/3  "<signal3>"
  Bus Selector/1 -> Data Store Write4/2  "<signal2>"
  Msg_Value_Data/1 -> Bus Selector/1
  Data Store Read/1 -> Cast17/1
  Cast8/1 -> Data Store Write5/1
  Cast9/1 -> Msg_Data_Encoder/2(tx_counter)
  Tx_ID/1 -> Cast8/1
  Cast17/1 -> Msg_Data_Encoder/3(verif_value)
  Data Store Read6/1 -> Cast18/1
  Msg_Data_Encoder/1(encoded_msg) -> Data Store Write4/1
  Data Store Read1/1 -> Cast9/1
  Cast18/1 -> Msg_Data_Encoder/1(basic_cycle)

== system HANcoder_E407_TTA_Controller_v4_5/HANcoder STM32 Target - E407-STM32 algorithm/TTA CAN System/TTA System/Matrix Cycle Manager/Vehicle Emulator Matrix Cycle/vehicle emulator basic cycle 0/COMM Task - Sync bc 0/Transmission subtasks/Msg_Value_Data_Encoded/float2uint1 ==
  precision : Inport
  magnitude : Inport  Port=2
  magnitude_max : Inport  Port=3
  magnitude_min : Inport  Port=4
  Abs : Abs
  Bit Shift : hdlsllib/Logic and Bit Operations/Bit Shift  mode=Shift Left Logical  N=7
      settings: SourceProductName=HDL Coder  SourceProductBaseCode=HD
  Cast : DataTypeConversion  OutDataTypeStr=uint8
  Cast1 : DataTypeConversion  OutDataTypeStr=uint8
  Cast2 : DataTypeConversion  OutDataTypeStr=uint8
  Constant : Constant  Value=0
  Constant1 : Constant  Value=2
  Constant2 : Constant  Value=2
  Divide : Product  Inputs=*/
  Fix : Rounding  Priority=3  Operator=fix
  Fix1 : Rounding  Priority=6  Operator=fix
  Gain : Gain  Gain=-1
  GreaterThan : RelationalOperator  Priority=2  Operator=<  OutDataTypeStr=boolean  RndMeth=Simplest
  LessThanOrEqual1 : RelationalOperator  OutDataTypeStr=boolean  RndMeth=Simplest
  LessThanOrEqual2 : RelationalOperator  Operator=<  OutDataTypeStr=boolean  RndMeth=Simplest
  Minus : Sum  Priority=4  Inputs=-+
  Multiply : Product
  Plus : Sum  Priority=10  Inputs=+++
  Power : Math  Priority=5  Operator=pow  SaturateOnIntegerOverflow=on
  Power1 : Math  Priority=5  Operator=pow  SaturateOnIntegerOverflow=on
  Switch : Switch  Criteria=u2 > Threshold
  Switch1 : Switch  Criteria=u2 > Threshold
  Switch2 : Switch  Criteria=u2 > Threshold
  coded : Outport
  wires:
  Switch1/1 -> Switch2/3
  Switch/1 -> Switch2/1
  LessThanOrEqual1/1 -> Switch1/2
  LessThanOrEqual2/1 -> Switch/2, Switch2/2
  magnitude_max/1 -> LessThanOrEqual2/1, Switch/1
  magnitude_min/1 -> Switch1/3, LessThanOrEqual1/2
  magnitude/1 -> Switch/3, LessThanOrEqual2/2, Switch1/1, LessThanOrEqual1/1
  Plus/1 -> coded/1
  [prec] -> Power1/2
  Multiply/1 -> Cast1/1
  precision/1 -> Gain/1, [prec]
  Power1/1 -> Multiply/2
  Constant2/1 -> Power1/1
  Cast2/1 -> Plus/3
  Fix1/1 -> Cast2/1
  Divide/1 -> Fix1/1
  Power/1 -> Divide/2
  Gain/1 -> Power/2
  Constant1/1 -> Power/1
  Cast1/1 -> Plus/2
  Bit Shift/1 -> Plus/1
  Cast/1 -> Bit Shift/1
  Minus/1 -> Divide/1
  Fix/1 -> Minus/1, Multiply/1
  GreaterThan/1 -> Cast/1
  Abs/1 -> Fix/1, Minus/2
  Switch2/1 -> GreaterThan/1, Abs/1
  Constant/1 -> GreaterThan/2

== system HANcoder_E407_TTA_Controller_v4_5/HANcoder STM32 Target - E407-STM32 algorithm/TTA CAN System/TTA System/Matrix Cycle Manager/Vehicle Emulator Matrix Cycle/vehicle emulator basic cycle 0/COMM Task - Sync bc 0/Transmission subtasks/Msg_Value_Data_Encoded/float2uint2 ==
  precision : Inport
  magnitude : Inport  Port=2
  magnitude_max : Inport  Port=3
  magnitude_min : Inport  Port=4
  Abs : Abs
  Bit Shift : hdlsllib/Logic and Bit Operations/Bit Shift  mode=Shift Left Logical  N=7
      settings: SourceProductName=HDL Coder  SourceProductBaseCode=HD
  Cast : DataTypeConversion  OutDataTypeStr=uint8
  Cast1 : DataTypeConversion  OutDataTypeStr=uint8
  Cast2 : DataTypeConversion  OutDataTypeStr=uint8
  Constant : Constant  Value=0
  Constant1 : Constant  Value=2
  Constant2 : Constant  Value=2
  Divide : Product  Inputs=*/
  Fix : Rounding  Priority=3  Operator=fix
  Fix1 : Rounding  Priority=6  Operator=fix
  Gain : Gain  Gain=-1
  GreaterThan : RelationalOperator  Priority=2  Operator=<  OutDataTypeStr=boolean  RndMeth=Simplest
  LessThanOrEqual1 : RelationalOperator  OutDataTypeStr=boolean  RndMeth=Simplest
  LessThanOrEqual2 : RelationalOperator  Operator=<  OutDataTypeStr=boolean  RndMeth=Simplest
  Minus : Sum  Priority=4  Inputs=-+
  Multiply : Product
  Plus : Sum  Priority=10  Inputs=+++
  Power : Math  Priority=5  Operator=pow  SaturateOnIntegerOverflow=on
  Power1 : Math  Priority=5  Operator=pow  SaturateOnIntegerOverflow=on
  Switch : Switch  Criteria=u2 > Threshold
  Switch1 : Switch  Criteria=u2 > Threshold
  Switch2 : Switch  Criteria=u2 > Threshold
  coded : Outport
  wires:
  Constant/1 -> GreaterThan/2
  Switch2/1 -> Abs/1, GreaterThan/1
  Abs/1 -> Minus/2, Fix/1
  GreaterThan/1 -> Cast/1
  Fix/1 -> Multiply/1, Minus/1
  Minus/1 -> Divide/1
  Cast/1 -> Bit Shift/1
  Bit Shift/1 -> Plus/1
  Cast1/1 -> Plus/2
  Constant1/1 -> Power/1
  Gain/1 -> Power/2
  Power/1 -> Divide/2
  Divide/1 -> Fix1/1
  Fix1/1 -> Cast2/1
  Cast2/1 -> Plus/3
  Constant2/1 -> Power1/1
  Power1/1 -> Multiply/2
  precision/1 -> [prec], Gain/1
  Multiply/1 -> Cast1/1
  [prec] -> Power1/2
  Plus/1 -> coded/1
  magnitude/1 -> LessThanOrEqual1/1, Switch1/1, LessThanOrEqual2/2, Switch/3
  magnitude_min/1 -> LessThanOrEqual1/2, Switch1/3
  magnitude_max/1 -> Switch/1, LessThanOrEqual2/1
  LessThanOrEqual2/1 -> Switch2/2, Switch/2
  LessThanOrEqual1/1 -> Switch1/2
  Switch/1 -> Switch2/1
  Switch1/1 -> Switch2/3

== system HANcoder_E407_TTA_Controller_v4_5/HANcoder STM32 Target - E407-STM32 algorithm/TTA CAN System/TTA System/Matrix Cycle Manager/Vehicle Emulator Matrix Cycle/vehicle emulator basic cycle 0/COMM Task - Sync bc 0/Transmission subtasks/Msg_Value_Data_Encoded/float2uint3 ==
  precision : Inport
  magnitude : Inport  Port=2
  magnitude_max : Inport  Port=3
  magnitude_min : Inport  Port=4
  Abs : Abs
  Bit Shift : hdlsllib/Logic and Bit Operations/Bit Shift  mode=Shift Left Logical  N=7
      settings: SourceProductName=HDL Coder  SourceProductBaseCode=HD
  Cast : DataTypeConversion  OutDataTypeStr=uint8
  Cast1 : DataTypeConversion  OutDataTypeStr=uint8
  Cast2 : DataTypeConversion  OutDataTypeStr=uint8
  Constant : Constant  Value=0
  Constant1 : Constant  Value=2
  Constant2 : Constant  Value=2
  Divide : Product  Inputs=*/
  Fix : Rounding  Priority=3  Operator=fix
  Fix1 : Rounding  Priority=6  Operator=fix
  Gain : Gain  Gain=-1
  GreaterThan : RelationalOperator  Priority=2  Operator=<  OutDataTypeStr=boolean  RndMeth=Simplest
  LessThanOrEqual1 : RelationalOperator  OutDataTypeStr=boolean  RndMeth=Simplest
  LessThanOrEqual2 : RelationalOperator  Operator=<  OutDataTypeStr=boolean  RndMeth=Simplest
  Minus : Sum  Priority=4  Inputs=-+
  Multiply : Product
  Plus : Sum  Priority=10  Inputs=+++
  Power : Math  Priority=5  Operator=pow  SaturateOnIntegerOverflow=on
  Power1 : Math  Priority=5  Operator=pow  SaturateOnIntegerOverflow=on
  Switch : Switch  Criteria=u2 > Threshold
  Switch1 : Switch  Criteria=u2 > Threshold
  Switch2 : Switch  Criteria=u2 > Threshold
  coded : Outport
  wires:
  Switch1/1 -> Switch2/3
  Switch/1 -> Switch2/1
  LessThanOrEqual1/1 -> Switch1/2
  LessThanOrEqual2/1 -> Switch/2, Switch2/2
  magnitude_max/1 -> LessThanOrEqual2/1, Switch/1
  magnitude_min/1 -> Switch1/3, LessThanOrEqual1/2
  magnitude/1 -> Switch/3, LessThanOrEqual2/2, Switch1/1, LessThanOrEqual1/1
  Plus/1 -> coded/1
  [prec] -> Power1/2
  Multiply/1 -> Cast1/1
  precision/1 -> Gain/1, [prec]
  Power1/1 -> Multiply/2
  Constant2/1 -> Power1/1
  Cast2/1 -> Plus/3
  Fix1/1 -> Cast2/1
  Divide/1 -> Fix1/1
  Power/1 -> Divide/2
  Gain/1 -> Power/2
  Constant1/1 -> Power/1
  Cast1/1 -> Plus/2
  Bit Shift/1 -> Plus/1
  Cast/1 -> Bit Shift/1
  Minus/1 -> Divide/1
  Fix/1 -> Minus/1, Multiply/1
  GreaterThan/1 -> Cast/1
  Abs/1 -> Fix/1, Minus/2
  Switch2/1 -> GreaterThan/1, Abs/1
  Constant/1 -> GreaterThan/2

== system HANcoder_E407_TTA_Controller_v4_5/HANcoder STM32 Target - E407-STM32 algorithm/TTA CAN System/TTA System/Matrix Cycle Manager/Vehicle Emulator Matrix Cycle/vehicle emulator basic cycle 0/COMM Task - Sync bc 0/Transmission subtasks/Msg_Value_Data_Encoded/float2uint4 ==
  precision : Inport
  magnitude : Inport  Port=2
  magnitude_max : Inport  Port=3
  magnitude_min : Inport  Port=4
  Abs : Abs
  Bit Shift : hdlsllib/Logic and Bit Operations/Bit Shift  mode=Shift Left Logical  N=7
      settings: SourceProductName=HDL Coder  SourceProductBaseCode=HD
  Cast : DataTypeConversion  OutDataTypeStr=uint8
  Cast1 : DataTypeConversion  OutDataTypeStr=uint8
  Cast2 : DataTypeConversion  OutDataTypeStr=uint8
  Constant : Constant  Value=0
  Constant1 : Constant  Value=2
  Constant2 : Constant  Value=2
  Divide : Product  Inputs=*/
  Fix : Rounding  Priority=3  Operator=fix
  Fix1 : Rounding  Priority=6  Operator=fix
  Gain : Gain  Gain=-1
  GreaterThan : RelationalOperator  Priority=2  Operator=<  OutDataTypeStr=boolean  RndMeth=Simplest
  LessThanOrEqual1 : RelationalOperator  OutDataTypeStr=boolean  RndMeth=Simplest
  LessThanOrEqual2 : RelationalOperator  Operator=<  OutDataTypeStr=boolean  RndMeth=Simplest
  Minus : Sum  Priority=4  Inputs=-+
  Multiply : Product
  Plus : Sum  Priority=10  Inputs=+++
  Power : Math  Priority=5  Operator=pow  SaturateOnIntegerOverflow=on
  Power1 : Math  Priority=5  Operator=pow  SaturateOnIntegerOverflow=on
  Switch : Switch  Criteria=u2 > Threshold
  Switch1 : Switch  Criteria=u2 > Threshold
  Switch2 : Switch  Criteria=u2 > Threshold
  coded : Outport
  wires:
  Constant/1 -> GreaterThan/2
  Switch2/1 -> Abs/1, GreaterThan/1
  Abs/1 -> Minus/2, Fix/1
  GreaterThan/1 -> Cast/1
  Fix/1 -> Multiply/1, Minus/1
  Minus/1 -> Divide/1
  Cast/1 -> Bit Shift/1
  Bit Shift/1 -> Plus/1
  Cast1/1 -> Plus/2
  Constant1/1 -> Power/1
  Gain/1 -> Power/2
  Power/1 -> Divide/2
  Divide/1 -> Fix1/1
  Fix1/1 -> Cast2/1
  Cast2/1 -> Plus/3
  Constant2/1 -> Power1/1
  Power1/1 -> Multiply/2
  precision/1 -> [prec], Gain/1
  Multiply/1 -> Cast1/1
  [prec] -> Power1/2
  Plus/1 -> coded/1
  magnitude/1 -> LessThanOrEqual1/1, Switch1/1, LessThanOrEqual2/2, Switch/3
  magnitude_min/1 -> LessThanOrEqual1/2, Switch1/3
  magnitude_max/1 -> Switch/1, LessThanOrEqual2/1
  LessThanOrEqual2/1 -> Switch2/2, Switch/2
  LessThanOrEqual1/1 -> Switch1/2
  Switch/1 -> Switch2/1
  Switch1/1 -> Switch2/3

== system HANcoder_E407_TTA_Controller_v4_5/HANcoder STM32 Target - E407-STM32 algorithm/TTA CAN System/TTA System/Matrix Cycle Manager/Vehicle Emulator Matrix Cycle/vehicle emulator basic cycle 0/COMM Task - Sync bc 0/Transmission subtasks/Msg_Value_Data_Encoded/float2uint8 ==
  precision : Inport
  magnitude : Inport  Port=2
  magnitude_max : Inport  Port=3
  magnitude_min : Inport  Port=4
  Abs : Abs
  Bit Shift : hdlsllib/Logic and Bit Operations/Bit Shift  mode=Shift Left Logical  N=7
      settings: SourceProductName=HDL Coder  SourceProductBaseCode=HD
  Cast : DataTypeConversion  OutDataTypeStr=uint8
  Cast1 : DataTypeConversion  OutDataTypeStr=uint8
  Cast2 : DataTypeConversion  OutDataTypeStr=uint8
  Constant : Constant  Value=0
  Constant1 : Constant  Value=2
  Constant2 : Constant  Value=2
  Divide : Product  Inputs=*/
  Fix : Rounding  Priority=3  Operator=fix
  Fix1 : Rounding  Priority=6  Operator=fix
  Gain : Gain  Gain=-1
  GreaterThan : RelationalOperator  Priority=2  Operator=<  OutDataTypeStr=boolean  RndMeth=Simplest
  LessThanOrEqual1 : RelationalOperator  OutDataTypeStr=boolean  RndMeth=Simplest
  LessThanOrEqual2 : RelationalOperator  Operator=<  OutDataTypeStr=boolean  RndMeth=Simplest
  Minus : Sum  Priority=4  Inputs=-+
  Multiply : Product
  Plus : Sum  Priority=10  Inputs=+++
  Power : Math  Priority=5  Operator=pow  SaturateOnIntegerOverflow=on
  Power1 : Math  Priority=5  Operator=pow  SaturateOnIntegerOverflow=on
  Switch : Switch  Criteria=u2 > Threshold
  Switch1 : Switch  Criteria=u2 > Threshold
  Switch2 : Switch  Criteria=u2 > Threshold
  coded : Outport
  wires:
  Constant/1 -> GreaterThan/2
  Switch2/1 -> Abs/1, GreaterThan/1
  Abs/1 -> Minus/2, Fix/1
  GreaterThan/1 -> Cast/1
  Fix/1 -> Multiply/1, Minus/1
  Minus/1 -> Divide/1
  Cast/1 -> Bit Shift/1
  Bit Shift/1 -> Plus/1
  Cast1/1 -> Plus/2
  Constant1/1 -> Power/1
  Gain/1 -> Power/2
  Power/1 -> Divide/2
  Divide/1 -> Fix1/1
  Fix1/1 -> Cast2/1
  Cast2/1 -> Plus/3
  Constant2/1 -> Power1/1
  Power1/1 -> Multiply/2
  precision/1 -> [prec], Gain/1
  Multiply/1 -> Cast1/1
  [prec] -> Power1/2
  Plus/1 -> coded/1
  magnitude/1 -> LessThanOrEqual1/1, Switch1/1, LessThanOrEqual2/2, Switch/3
  magnitude_min/1 -> LessThanOrEqual1/2, Switch1/3
  magnitude_max/1 -> Switch/1, LessThanOrEqual2/1
  LessThanOrEqual2/1 -> Switch2/2, Switch/2
  LessThanOrEqual1/1 -> Switch1/2
  Switch/1 -> Switch2/1
  Switch1/1 -> Switch2/3
